simulink model "taller2"  (Simulink 7.2)
settings: Solver=ode45  StartTime=0.0  StopTime=10.0  RelTol=1e-3
values from neighbouring files (symbols this model uses):
  Beq = 2.5821e-4    (= 0.00025821)    [GlobalParam.m]
  Jeq = 7.7463e-4    (= 0.00077463)    [GlobalParam.m]
  K = 0.06    [GlobalParam.m]
  L = 91.7e-3    (= 0.0917)    [GlobalParam.m]
  R = 19.8    [GlobalParam.m]
settings Model: Creator=ALan  LastModifiedBy=ALan

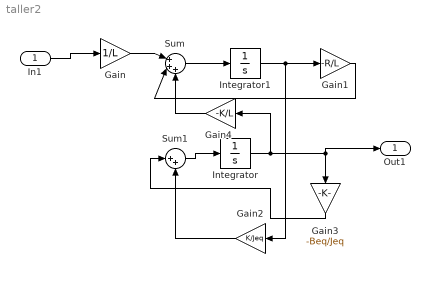
== system taller2 ==
  In1 : Inport  OutDataType=sfix(16)  OutScaling=2^0
  Gain : Gain  Gain=1/L  ParameterDataType=sfix(16)  ParameterScaling=2^0  OutDataType=sfix(16)  OutScaling=2^0
  Gain1 : Gain  Gain=-R/L  ParameterDataType=sfix(16)  ParameterScaling=2^0  OutDataType=sfix(16)  OutScaling=2^0
  Gain2 : Gain  Orientation=left  Gain=K/Jeq  ParameterDataType=sfix(16)  ParameterScaling=2^0  OutDataType=sfix(16)  OutScaling=2^0
  Gain3 : Gain  Orientation=down  Gain=-Beq/Jeq  ParameterDataType=sfix(16)  ParameterScaling=2^0  OutDataType=sfix(16)  OutScaling=2^0
  Gain4 : Gain  Orientation=left  Gain=-K/L  ParameterDataType=sfix(16)  ParameterScaling=2^0  OutDataType=sfix(16)  OutScaling=2^0
  Integrator : Integrator
  Integrator1 : Integrator
  Sum : Sum  Inputs=|+++  OutDataType=sfix(16)  OutScaling=2^0
  Sum1 : Sum  Inputs=|++  OutDataType=sfix(16)  OutScaling=2^0
  Out1 : Outport  OutDataType=sfix(16)  OutScaling=2^0
  wires:
  Gain/1 -> Sum/1
  In1/1 -> Gain/1
  Sum/1 -> Integrator1/1
  Integrator1/1 -> Gain1/1, Gain2/1
  Gain1/1 -> Sum/2
  Sum1/1 -> Integrator/1
  Gain2/1 -> Sum1/2
  Integrator/1 -> Gain3/1, Out1/1, Gain4/1
  Gain3/1 -> Sum1/1
  Gain4/1 -> Sum/3
